simulink model "AC_DC_Converter"  (R2015a)
settings: Solver=ode45  StartTime=0.0  StopTime=0.1  RelTol=1e-3
libraries: powerlib x1
settings Model: Creator=Koustubh  LastModifiedBy=Koustubh

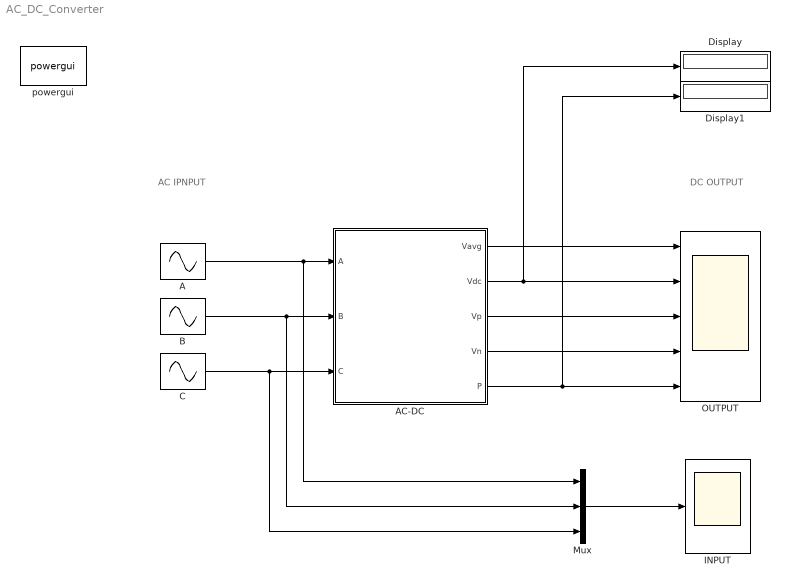
== system AC_DC_Converter ==
  note: DC OUTPUT
  note: AC IPNPUT
  A : Sin  Amplitude=230  Frequency=2*pi*60  SampleTime=0
  AC-DC : Subsystem
  B : Sin  Amplitude=230  Frequency=2*pi*60  Phase=2*pi/3  SampleTime=0
  C : Sin  Amplitude=230  Frequency=2*pi*60  Phase=4*pi/3  SampleTime=0
  Display : Display
  Display1 : Display
  INPUT : Scope
  Mux : Mux  Inputs=3
  OUTPUT : Scope  NumInputPorts=5
      settings: YMin=-5~-5~-5~-5~-5  YMax=5~5~5~5~5
  powergui : powerlib/powergui  Priority=1  SimulationMode=Discrete  SolverType=Tustin/Backward Euler (TBE)  SampleTime=50e-6  frequency=60  SPID=off  DisableSnubberDevices=off  DisableRonSwitches=off  DisableVfSwitches=off  SwTol=0  DisplayEquations=off  Interpol=off  methode=off  Ts=100  FunctionMessages=off  echomessages=off  HookPort=off  EnableUseOfTLC=off  x0status=blocks  frequencyindice=60  Pbase=100e6  ErrMax=1e-4  Iterations=50  UnitsV=kV  UnitsW=MW  buscounter=0  RestoreLinks=warning  ResistiveCurrentMeasurement=off  Frange=[0:2:500]  Ylog=off  Xlog=on  ShowGrid=off  save=off  variable=ZData  structure=0  ZoomFFT=off  StartTime=0.0  cycles=1  DisplayStyle=1  fundamental=60  FreqAxis=off  MaxFrequency=1000  frequencyindicesteady=1  RmsSteady=1  display=off
  wires:
  B/1 -> Mux/2, AC-DC/2(B)
  A/1 -> Mux/1, AC-DC/1(A)
  C/1 -> Mux/3, AC-DC/3(C)
  AC-DC/1(Vavg) -> OUTPUT/1
  AC-DC/2(Vdc) -> Display/1, OUTPUT/2
  AC-DC/3(Vp) -> OUTPUT/3
  AC-DC/4(Vn) -> OUTPUT/4
  Mux/1 -> INPUT/1
  AC-DC/5(P) -> Display1/1, OUTPUT/5

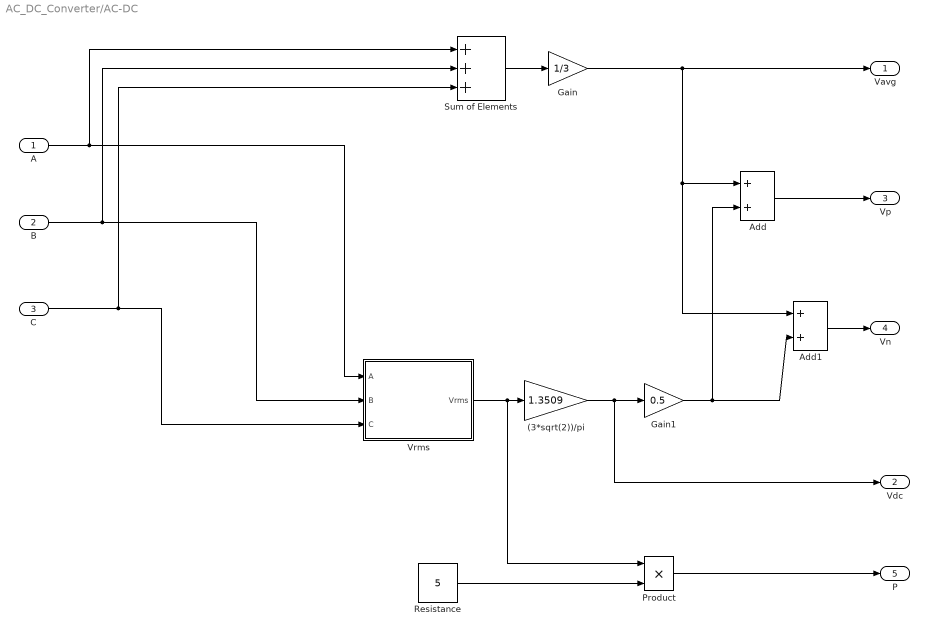
== system AC_DC_Converter/AC-DC ==
  A : Inport
  B : Inport  Port=2
  C : Inport  Port=3
  (3*sqrt(2))/pi : Gain  Gain=1.3509
  Add : Sum
  Add1 : Sum
  Gain : Gain  Gain=1/3
  Gain1 : Gain  Gain=0.5
  Product : Product
  Resistance : Constant  Value=5
  Sum of Elements : Sum  Inputs=+++
  Vrms : Subsystem
  Vavg : Outport
  Vdc : Outport  Port=2
  Vp : Outport  Port=3
  Vn : Outport  Port=4
  P : Outport  Port=5
  wires:
  A/1 -> Sum of Elements/1, Vrms/1(A)
  B/1 -> Sum of Elements/2, Vrms/2(B)
  C/1 -> Sum of Elements/3, Vrms/3(C)
  Sum of Elements/1 -> Gain/1
  Gain/1 -> Add1/1, Add/1, Vavg/1
  Vrms/1(Vrms) -> Product/1, (3*sqrt(2))/pi/1
  (3*sqrt(2))/pi/1 -> Vdc/1, Gain1/1
  Gain1/1 -> Add/2, Add1/2
  Add1/1 -> Vn/1
  Add/1 -> Vp/1
  Resistance/1 -> Product/2
  Product/1 -> P/1

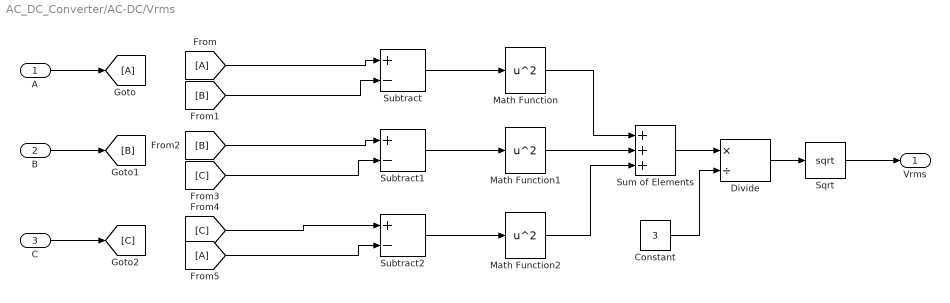
== system AC_DC_Converter/AC-DC/Vrms ==
  A : Inport
  B : Inport  Port=2
  C : Inport  Port=3
  Constant : Constant  Value=3
  Divide : Product  Inputs=*/
  Math Function : Math  Operator=square  SaturateOnIntegerOverflow=on
  Math Function1 : Math  Operator=square  SaturateOnIntegerOverflow=on
  Math Function2 : Math  Operator=square  SaturateOnIntegerOverflow=on
  Sqrt : Sqrt  SaturateOnIntegerOverflow=on
  Subtract : Sum  Inputs=+-
  Subtract1 : Sum  Inputs=+-
  Subtract2 : Sum  Inputs=+-
  Sum of Elements : Sum  Inputs=+++
  Vrms : Outport
  wires:
  Sqrt/1 -> Vrms/1
  B/1 -> [B]
  C/1 -> [C]
  A/1 -> [A]
  Divide/1 -> Sqrt/1
  Sum of Elements/1 -> Divide/1
  Constant/1 -> Divide/2
  [A] -> Subtract/1
  [B] -> Subtract1/1
  [B] -> Subtract/2
  [A] -> Subtract2/2
  [C] -> Subtract1/2
  [C] -> Subtract2/1
  Math Function1/1 -> Sum of Elements/2
  Subtract2/1 -> Math Function2/1
  Math Function/1 -> Sum of Elements/1
  Subtract/1 -> Math Function/1
  Math Function2/1 -> Sum of Elements/3
  Subtract1/1 -> Math Function1/1
